simulink model "FECG_hdl_fix1"  (Simulink 7.8)
settings: Solver=FixedStepDiscrete  SolverMode=SingleTasking  StartTime=0.0  StopTime=60  RelTol=1e-3
PreLoadFcn:
  | mom_and_fetus;
InitFcn:
  | num = fir1(1000,100/4000); %'FIR (all zeros)'
libraries: dspsrcs4 x2, dsparch4 x1, dspadpt3 x1
settings Model: MinMaxOverflowLogging=MinMaxAndOverflow  Creator=igal  LastModifiedBy=igal
settings SolverCC: PositivePriorityOrder=on
settings OptimizationCC: BlockReduction=off  ConditionallyExecuteInputs=off
settings DebuggingCC: FcnCallInpInsideContextMsg=Use local settings

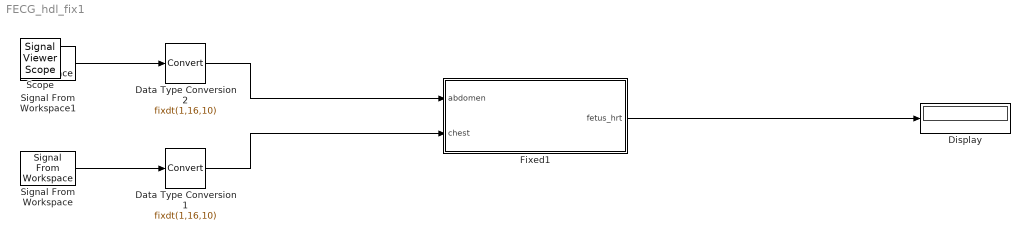
== system FECG_hdl_fix1 ==
  Data Type Conversion1 : DataTypeConversion  OutDataTypeStr=fixdt(1,16,10)  SaturateOnIntegerOverflow=on
  Data Type Conversion2 : DataTypeConversion  OutDataTypeStr=fixdt(1,16,10)  SaturateOnIntegerOverflow=on
  Display : Display
  Fixed1 : Subsystem  MinMaxOverflowLogging=MinMaxAndOverflow
  Signal From Workspace : dspsrcs4/Signal From Workspace  X=x  Ts=1/4e3  nsamps=1  OutputAfterFinalValue=Cyclic repetition  ignoreOrWarnInputAndFrameLengths=off
  Signal From Workspace1 : dspsrcs4/Signal From Workspace  X=d  Ts=1/4e3  nsamps=1  OutputAfterFinalValue=Cyclic repetition  ignoreOrWarnInputAndFrameLengths=off
  Scope : SignalViewerScope  IOType=viewer  RefreshTime=0.035000
      settings: TickLabels=off  YMin=0  YMax=190
  wires:
  Signal From Workspace1/1 -> Data Type Conversion2/1
  Signal From Workspace/1 -> Data Type Conversion1/1
  Fixed1/1(fetus_hrt) -> Display/1
  Data Type Conversion2/1 -> Fixed1/1(abdomen)
  Data Type Conversion1/1 -> Fixed1/2(chest)

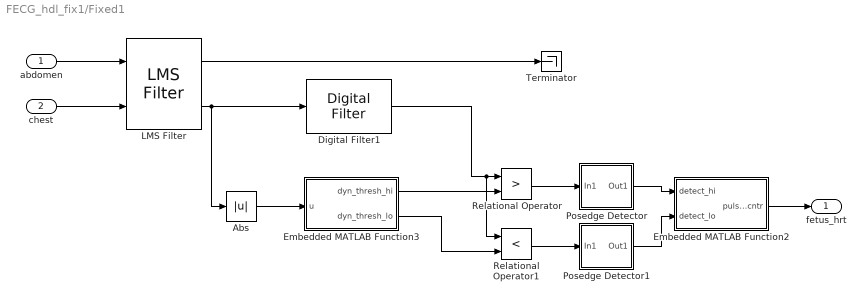
== system FECG_hdl_fix1/Fixed1 ==
  abdomen : Inport
  chest : Inport  Port=2
  Abs : Abs
  Digital Filter1 : dsparch4/Digital Filter  TypePopup=FIR (all zeros)  IIRFiltStruct=Direct form I transposed  AllPoleFiltStruct=Direct form  FIRFiltStruct=Direct form  CoeffSource=Specify via dialog  NumCoeffs=num  DenCoeffs=den  BiQuadCoeffs=[1 0.3 0.4 1 0.1 0.2]  LatticeCoeffs=[0.2 0.4]  denIgnore=on  FiltPerSampPopup=One filter per frame  IC=0  ICnum=0  ICden=0  firstCoeffMode=Binary point scaling  firstCoeffWordLength=16  firstCoeffFracLength=15  accumMode=Binary point scaling  accumWordLength=32  accumFracLength=30  prodOutputMode=Binary point scaling  prodOutputWordLength=32  prodOutputFracLength=30  roundingMode=Floor  overflowMode=off  ScaleValues=1  scaleValueFracLength=14  stageInFracLength=15  stageOutFracLength=15  FilterSource=Specify via dialog  dfiltObjectName=Hd  InputProcessing=Inherited (this choice will be removed - see release notes)
  Embedded MATLAB Function2 : MATLAB Function  TreatAsAtomicUnit=on
  Embedded MATLAB Function3 : MATLAB Function  TreatAsAtomicUnit=on
  LMS Filter : dspadpt3/LMS Filter  Algo=LMS  L=15  stepflag=Dialog  mu=0.001  leakage=1  ic=0  Adapt=off  resetflag=None  weights=off  firstCoeffMode=Binary point scaling  firstCoeffWordLength=32  firstCoeffFracLength=31  secondCoeffMode=User-defined  secondCoeffWordLength=2  secondCoeffFracLength=31  accumMode=Binary point scaling  accumWordLength=32  accumFracLength=20  accum2Mode=User-defined  accum2FracLength=20  prodOutputMode=Binary point scaling  prodOutputWordLength=32  prodOutputFracLength=20  prodOutput2Mode=User-defined  prodOutput2FracLength=30  prodOutput3Mode=User-defined  prodOutput3FracLength=30  prodOutput4Mode=User-defined  prodOutput4FracLength=30  quotientMode=User-defined  quotientFracLength=20  memoryMode=Binary point scaling  memoryWordLength=32  memoryFracLength=31  roundingMode=Floor  overflowMode=off  addnparflag=off
  Posedge Detector : Subsystem
      mask Display: disp('Posedge\n Detect');
  Posedge Detector1 : Subsystem
      mask Display: disp('Posedge\n Detect');
  Relational Operator : RelationalOperator  Operator=>  OutDataTypeStr=boolean
  Relational Operator1 : RelationalOperator  Operator=<  OutDataTypeStr=boolean
  Terminator : Terminator
  fetus_hrt : Outport
  wires:
  LMS Filter/2 -> Digital Filter1/1, Abs/1
  Digital Filter1/1 -> Relational Operator/1, Relational Operator1/1
  Abs/1 -> Embedded MATLAB Function3/1(u)
  Relational Operator/1 -> Posedge Detector/1(In1)
  abdomen/1 -> LMS Filter/1
  chest/1 -> LMS Filter/2
  LMS Filter/1 -> Terminator/1
  Embedded MATLAB Function2/1(pulse_cntr) -> fetus_hrt/1
  Posedge Detector/1(Out1) -> Embedded MATLAB Function2/1(detect_hi)
  Relational Operator1/1 -> Posedge Detector1/1(In1)
  Posedge Detector1/1(Out1) -> Embedded MATLAB Function2/2(detect_lo)
  Embedded MATLAB Function3/1(dyn_thresh_hi) -> Relational Operator/2
  Embedded MATLAB Function3/2(dyn_thresh_lo) -> Relational Operator1/2

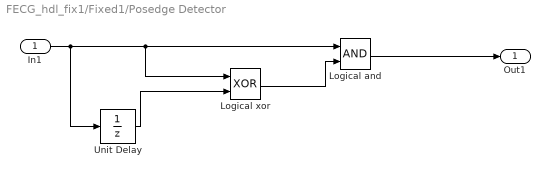
== system FECG_hdl_fix1/Fixed1/Posedge Detector ==
  In1 : Inport
  Logical and : Logic  AllPortsSameDT=off  OutDataTypeStr=boolean
  Logical xor : Logic  Operator=XOR  AllPortsSameDT=off  OutDataTypeStr=boolean
  Unit Delay : UnitDelay  SampleTime=-1
  Out1 : Outport
  wires:
  Logical and/1 -> Out1/1
  In1/1 -> Unit Delay/1, Logical xor/1, Logical and/1
  Logical xor/1 -> Logical and/2
  Unit Delay/1 -> Logical xor/2

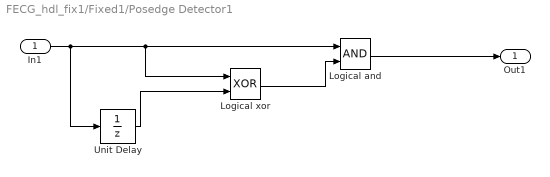
== system FECG_hdl_fix1/Fixed1/Posedge Detector1 ==
  In1 : Inport
  Logical and : Logic  AllPortsSameDT=off  OutDataTypeStr=boolean
  Logical xor : Logic  Operator=XOR  AllPortsSameDT=off  OutDataTypeStr=boolean
  Unit Delay : UnitDelay  SampleTime=-1
  Out1 : Outport
  wires:
  Unit Delay/1 -> Logical xor/2
  Logical xor/1 -> Logical and/2
  In1/1 -> Logical and/1, Logical xor/1, Unit Delay/1
  Logical and/1 -> Out1/1

== matlab function Fixed1/Embedded MATLAB Function2 ==
  data: detect_hi input double; pulse_cntr output double; detect_lo input double
function pulse_cntr = fcn(detect_hi, detect_lo) %#codegen
%Moving average, implemented with circular buffer
avg_length = 20e3;
persistent indx;
persistent sigma_hi;
persistent buffer_hi;
persistent sigma_lo;
persistent buffer_lo;

if isempty(indx)
    indx = 1;
    sigma_hi = int16(0);
    sigma_lo = int16(0);
    buffer_hi = false(1,avg_length);
    buffer_lo = false(1,avg_length);
end
sigma_hi = int16(sigma_hi - int16(buffer_hi(indx)));
sigma_lo = int16(sigma_lo - int16(buffer_lo(indx)));
buffer_hi(indx) = detect_hi;
buffer_lo(indx) = detect_lo;
sigma_hi = int16(sigma_hi + int16(buffer_hi(indx)));
sigma_lo = int16(sigma_lo + int16(buffer_lo(indx)));

%indx = mod(indx,avg_length)+1;
if (indx == avg_length)
    indx = 1;
else
    indx = indx + 1;
end

pulse_cntr = int16((sigma_hi+sigma_lo) * 6);

== matlab function Fixed1/Embedded MATLAB Function3 ==
  data: u input double; dyn_thresh_hi output double; dyn_thresh_lo output double
function [dyn_thresh_hi, dyn_thresh_lo] = fcn(u) %#codegen
%Moving average, implemented with circular buffer
avg_length = 8192;
thresh_gain = 3;
persistent indx;
persistent sigma;
persistent buffer;
persistent dvalid;
if isempty(indx)
    indx = 1;
    sigma = fi(0,1,32,10);
    buffer = fi(zeros(1,avg_length),1,16,10);
    dvalid = false;
end
sigma = fi(sigma - buffer(indx),1,32,10);
buffer(indx) = u;
sigma = fi(sigma + buffer(indx),1,32,10);

%indx = mod(indx,avg_length)+1;
if (indx == avg_length)
    indx = 1;
else
    indx = indx + 1;
end

if (indx >= avg_length)
    dvalid = true;
end

if (dvalid)
    sub_thresh = thresh_gain*sigma/avg_length;
    dyn_thresh_hi = fi(sub_thresh,1,16,10);
    dyn_thresh_lo = fi(-sub_thresh,1,16,10);
else
    dyn_thresh_hi = fi(0.5,1,16,10);
    dyn_thresh_lo = fi(-0.5,1,16,10);
end
